simulink library "Weather_from_File"  (Simulink 8.2)
settings: Solver=ode45  StartTime=0.0  StopTime=10.0  RelTol=1e-3
undefined symbols (not defined in the file): t_sample
libraries: carnot x1
settings Model: Creator=lena.frank  LastModifiedBy=drhf

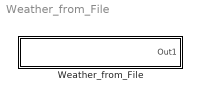
== system Weather_from_File ==
  Weather_from_File : Subsystem  mask(weather from file){file=DE_TRY2010_04_averageYear, ext=.mat}
      mask prompts: file "Name of file"; ext "Extension of file"
      mask help:
      | Input block for external weather data files. The file is read to the workspace. A "From Workspace" Block is used in the subsystem.
      | A Unit-Delay with the timestep of the weather data forces the model to a maximum timestep equal to the data acquisiton timestep.
      | Remark: Be carefull when using the TRY Data 2010 for Germany. The files are public and can be found in the parameter_set folder of this block. But there are bugs is the solar radiation data.
      mask init:
      | % path definitions
      | parampath = fullfile('Weather','Weather_from_File','parameter_set');
      | 
      | CarnotCallbacks_GetFiles;
      | 
      | % filename = [file, ext];
      | % intfile = fullfile(path_carnot('intlibsl'), parampath, filename);
      | % pubfile = fullfile(path_carnot('libsl'), parampath, filename);
      | % 
      | % if ~BlockIsInCarnotLibrary          % not in carnot library any more
      | %     if exist(filename,'file')       % search file on matlab path
      | %         evalin('base',['load(''' filename ''');'])
      | %     elseif exist(intfile,'file')    % search on internal path
      | %         evalin('base',['load(''' intfile ''');'])
      | %     elseif exist(pubfile,'file')    % search on public path
      | %         evalin('base',['load(''' pubfile ''');'])
      | %     end
      | %     set_param([gcb '/From_Workspace'], 'VariableName', file);
      | % end
      | % 
      | % % sample time is timestep of weather data
      | % rawdata = load(file);
      | % varnames = fieldnames(rawdata);
      | % t_sample = rawdata.(varnames{1})(3,1) - rawdata.(varnames{1})(2,1);
      | % clear rawdata;
      | % clear varnames;
      mask Help: web(fullfile(path_carnot('help'),'weather_from_file.html'),'-helpbrowser')
      mask TypeOptions ext: .dat | .txt | .mat
      mask Display: disp(file)

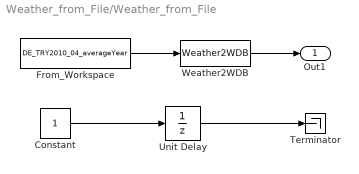
== system Weather_from_File/Weather_from_File ==
  Constant : Constant
  From_Workspace : FromWorkspace  VariableName=DE_TRY2010_04_averageYear  SampleTime=0  OutputAfterFinalValue=Setting to zero
  Terminator : Terminator
  Unit Delay : UnitDelay  SampleTime=t_sample
  Weather2WDB : carnot/Toolbox/Weather2WDB
  Out1 : Outport
  wires:
  From_Workspace/1 -> Weather2WDB/1
  Constant/1 -> Unit Delay/1
  Unit Delay/1 -> Terminator/1
  Weather2WDB/1 -> Out1/1
